simulink model "controller1"  (R2017b)
settings: Solver=VariableStepAuto  StartTime=0.0  StopTime=10.0  RelTol=1e-3
values from neighbouring files (symbols this model uses):
  d = 0.15    [extendedKalman.m]    (also in extendedKalmanFilter.m; plant.m = 0.24; runV3.m; runpathfollower.m)
  dt = 0.1    [extendedKalmanFilter.m]    (also in matlab.mat; runV3.m; rungen.m; runpathfollower.m)
  k1 = 8    [runpathfollower.m]    (also in runpathplanner.m = 1)
  k2 = 1    [runpathfollower.m]    (also in runpathplanner.m)
  theta_mi = 30*pi/180    (= 0.523598775598)    [runpathfollower.m]    (also in runpathplanner.m = 0.785398163397)
  xi = 1.5    [runpathfollower.m]    (also in runpathplanner.m = 0)
  yi = 2.3    [runpathfollower.m]    (also in runpathplanner.m = 1.5)
undefined symbols (not defined in the file or in its folder): DiscIntNeverNeededParam, gamma, radius, theta_a
settings Model: Creator=nisha  LastModifiedBy=nisha

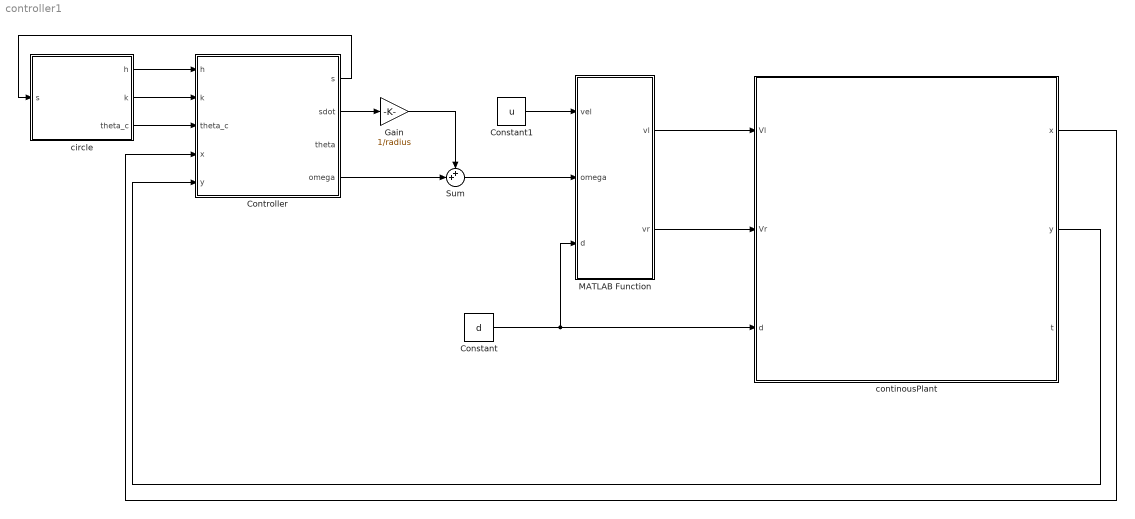
== system controller1 ==
  Constant : Constant  Value=d
  Constant1 : Constant  Value=u
  Controller : Subsystem
  Gain : Gain  Gain=1/radius
  MATLAB Function : MATLAB Function  TreatAsAtomicUnit=on
  Sum : Sum  Inputs=++|
  circle : Subsystem
  continousPlant : Subsystem  TreatAsAtomicUnit=on
  wires:
  MATLAB Function/2(vr) -> continousPlant/2(Vr)
  MATLAB Function/1(vl) -> continousPlant/1(Vl)
  Constant/1 -> MATLAB Function/3(d), continousPlant/3(d)
  circle/1(h) -> Controller/1(h)
  circle/2(k) -> Controller/2(k)
  circle/3(theta_c) -> Controller/3(theta_c)
  Controller/1(s) -> circle/1(s)
  continousPlant/1(x) -> Controller/4(x)
  continousPlant/2(y) -> Controller/5(y)
  Controller/4(omega) -> Sum/2
  Gain/1 -> Sum/1
  Controller/2(sdot) -> Gain/1
  Sum/1 -> MATLAB Function/2(omega)
  Constant1/1 -> MATLAB Function/1(vel)

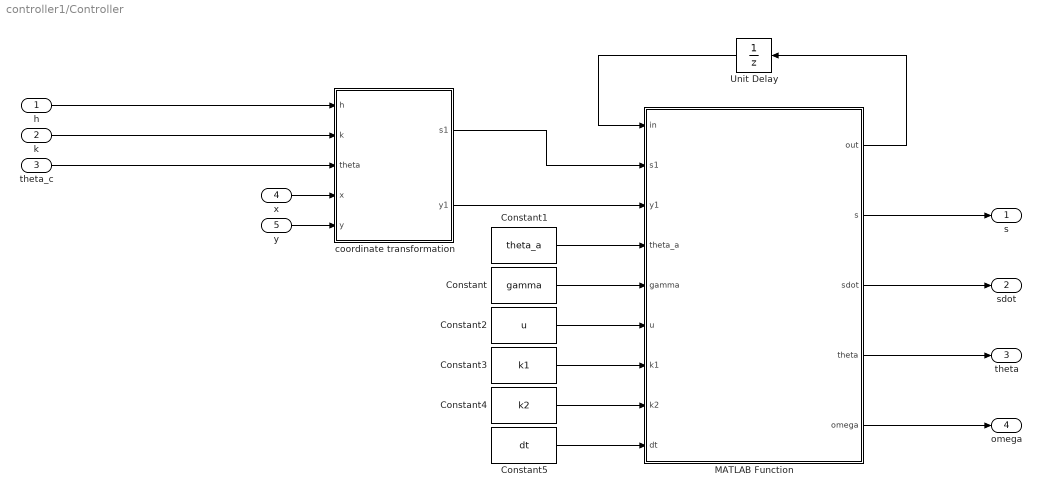
== system controller1/Controller ==
  h : Inport
  k : Inport  Port=2
  theta_c : Inport  Port=3
  x : Inport  Port=4
  y : Inport  Port=5
  Constant : Constant  Value=gamma
  Constant1 : Constant  Value=theta_a
  Constant2 : Constant  Value=u
  Constant3 : Constant  Value=k1
  Constant4 : Constant  Value=k2
  Constant5 : Constant  Value=dt
  MATLAB Function : MATLAB Function  TreatAsAtomicUnit=on
  Unit Delay : UnitDelay  InitialCondition=[0,0,theta_mi,0]'  SampleTime=-1
  coordinate transformation : Subsystem
  s : Outport
  sdot : Outport  Port=2
  theta : Outport  Port=3
  omega : Outport  Port=4
  wires:
  MATLAB Function/1(out) -> Unit Delay/1
  Unit Delay/1 -> MATLAB Function/1(in)
  coordinate transformation/1(s1) -> MATLAB Function/2(s1)
  coordinate transformation/2(y1) -> MATLAB Function/3(y1)
  Constant/1 -> MATLAB Function/5(gamma)
  Constant2/1 -> MATLAB Function/6(u)
  Constant3/1 -> MATLAB Function/7(k1)
  Constant4/1 -> MATLAB Function/8(k2)
  Constant5/1 -> MATLAB Function/9(dt)
  MATLAB Function/2(s) -> s/1
  MATLAB Function/4(theta) -> theta/1
  y/1 -> coordinate transformation/5(y)
  x/1 -> coordinate transformation/4(x)
  theta_c/1 -> coordinate transformation/3(theta)
  k/1 -> coordinate transformation/2(k)
  h/1 -> coordinate transformation/1(h)
  MATLAB Function/5(omega) -> omega/1
  MATLAB Function/3(sdot) -> sdot/1
  Constant1/1 -> MATLAB Function/4(theta_a)

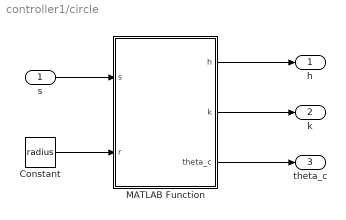
== system controller1/circle ==
  s : Inport
  Constant : Constant  Value=radius
  MATLAB Function : MATLAB Function  TreatAsAtomicUnit=on
  h : Outport
  k : Outport  Port=2
  theta_c : Outport  Port=3
  wires:
  s/1 -> MATLAB Function/1(s)
  Constant/1 -> MATLAB Function/2(r)
  MATLAB Function/1(h) -> h/1
  MATLAB Function/2(k) -> k/1
  MATLAB Function/3(theta_c) -> theta_c/1

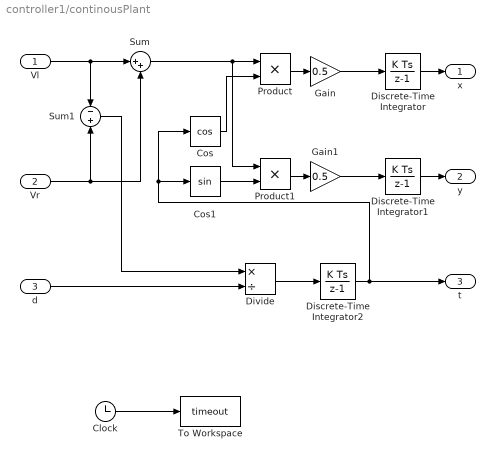
== system controller1/continousPlant ==
  Vl : Inport
  Vr : Inport  Port=2
  d : Inport  Port=3
  Clock : Clock
  Cos : Trigonometry  Operator=cos
  Cos1 : Trigonometry
  Discrete-Time Integrator : DiscreteIntegrator  InitialCondition=xi  InitialConditionSetting=State (most efficient)  SampleTime=-1  ICPrevOutput=DiscIntNeverNeededParam  ICPrevScaledInput=DiscIntNeverNeededParam
  Discrete-Time Integrator1 : DiscreteIntegrator  InitialCondition=yi  InitialConditionSetting=State (most efficient)  SampleTime=-1  ICPrevOutput=DiscIntNeverNeededParam  ICPrevScaledInput=DiscIntNeverNeededParam
  Discrete-Time Integrator2 : DiscreteIntegrator  InitialCondition=theta_mi  InitialConditionSetting=State (most efficient)  SampleTime=-1  ICPrevOutput=DiscIntNeverNeededParam  ICPrevScaledInput=DiscIntNeverNeededParam
  Divide : Product  Inputs=*/
  Gain : Gain  Gain=0.5
  Gain1 : Gain  Gain=0.5
  Product : Product
  Product1 : Product
  Sum : Sum  Inputs=|++
  Sum1 : Sum  Inputs=-|+
  To Workspace : ToWorkspace  VariableName=timeout  SampleTime=-1
  x : Outport
  y : Outport  Port=2
  t : Outport  Port=3
  wires:
  Vl/1 -> Sum/1, Sum1/1
  Vr/1 -> Sum/2, Sum1/2
  Sum/1 -> Product1/1, Product/1
  Product1/1 -> Gain1/1
  Product/1 -> Gain/1
  Gain1/1 -> Discrete-Time Integrator1/1
  d/1 -> Divide/2
  Divide/1 -> Discrete-Time Integrator2/1
  Sum1/1 -> Divide/1
  Cos/1 -> Product/2
  Cos1/1 -> Product1/2
  Discrete-Time Integrator2/1 -> t/1, Cos1/1, Cos/1
  Discrete-Time Integrator1/1 -> y/1
  Gain/1 -> Discrete-Time Integrator/1
  Clock/1 -> To Workspace/1
  Discrete-Time Integrator/1 -> x/1

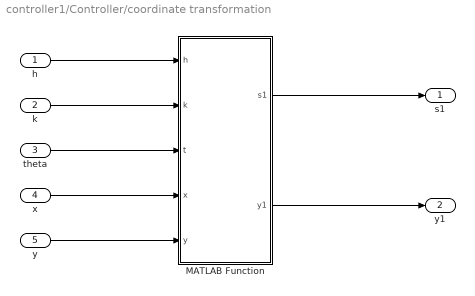
== system controller1/Controller/coordinate transformation ==
  h : Inport
  k : Inport  Port=2
  theta : Inport  Port=3
  x : Inport  Port=4
  y : Inport  Port=5
  MATLAB Function : MATLAB Function  TreatAsAtomicUnit=on
  s1 : Outport
  y1 : Outport  Port=2
  wires:
  theta/1 -> MATLAB Function/3(t)
  k/1 -> MATLAB Function/2(k)
  h/1 -> MATLAB Function/1(h)
  x/1 -> MATLAB Function/4(x)
  y/1 -> MATLAB Function/5(y)
  MATLAB Function/1(s1) -> s1/1
  MATLAB Function/2(y1) -> y1/1

== matlab function controller1/Controller/coordinate transformation/MATLAB Function ==
  data: h input; s1 output; k input; t input; x input; y input; y1 output
function [s1,y1] = fcn(h,k,t,x,y)
A=[cos(t) sin(t)
  -sin(t) cos(t)];
X = A*[x-h y-k]';
s1=X(1);
y1=X(2);

== matlab function controller1/MATLAB Function ==
  data: vel input; vl output; omega input; d input; vr output
function [vl, vr] = fcn(vel, omega,d)
vr=vel +d/2*omega;
vl=vel -d/2*omega;
end

== matlab function controller1/Controller/MATLAB Function ==
  data: in input; s1 input; y1 input; theta_a input; gamma input; u input; out output; k1 input; k2 input; dt input; s output; sdot output; theta output; omega output
function [out,s,sdot,theta,omega] = fcn(in,s1,y1,theta_a,gamma,u,k1,k2,dt)
delta=-sign(u)*theta_a*tanh(y1);
out=[in(1)+(u*cos(in(2))+k1*s1)*dt;
     u*cos(in(2))+k1*s1
     in(2)+(-gamma*y1*u*(sin(in(2))-sin(delta))/(in(2)-delta)-k2*(in(2)-delta))*dt
     -gamma*y1*u*(sin(in(2))-sin(delta))/(in(2)-delta)-k2*(in(2)-delta)];
s=out(1); sdot=out(2); theta=out(3); omega=out(4);

== matlab function controller1/circle/MATLAB Function ==
  data: s input; h output; r input; k output; theta_c output
function [h,k,theta_c] = fcn(s,r)
h=r*cos(s/r);
k=r*sin(s/r);
theta_c=-1/tan(s/r);
